simulink model "InvPend"  (Simulink 7.6)
settings: Solver=ode4  StartTime=0.0  StopTime=20  FixedStep=0.01  RelTol=1e-3
values from neighbouring files (symbols this model uses):
  c = 6/(7*l + (b^2)/l)    (= 1.71389396709)    [MasterP_4DInvPendData_BEST.m]    (also in MasterP_4DInvPendData_MAIN.m)
  g = 9.81    [MasterP_4DInvPendData_BEST.m]    (also in MasterP_4DInvPendData_MAIN.m)
  kP = 1    [MasterP_4DInvPendData_BEST.m]    (also in MasterP_4DInvPendData_MAIN.m)
  T1 = 0.0395    [MasterP_4DInvPendData_BEST.m]    (also in MasterP_4DInvPendData_MAIN.m)
undefined symbols (not defined in the file or in its folder): SU
settings Model: Creator=Mohsen  LastModifiedBy=Mohsen

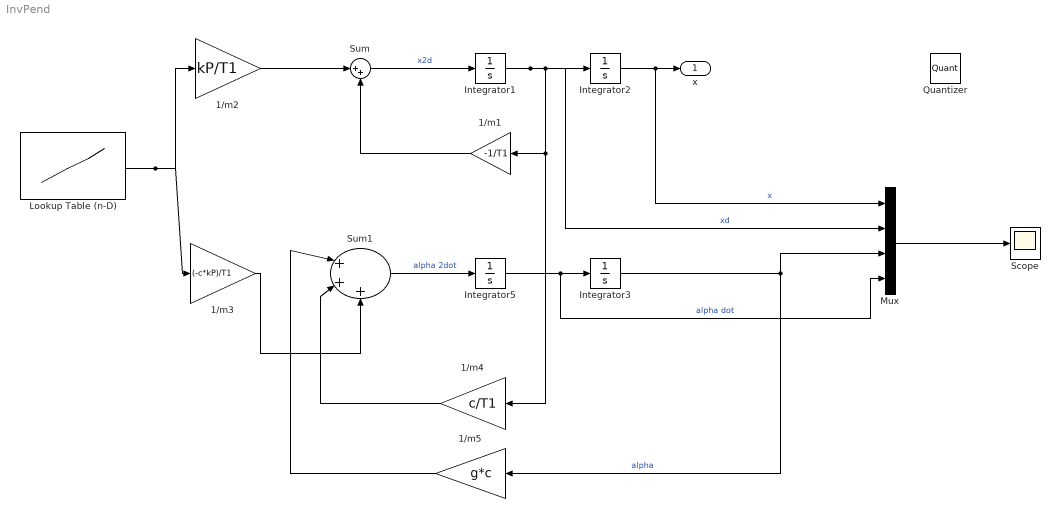
== system InvPend ==
  1/m1 : Gain  Gain=-1/T1
  1/m2 : Gain  Gain=kP/T1
  1/m3 : Gain  Gain=(-c*kP)/T1
  1/m4 : Gain  Gain=c/T1
  1/m5 : Gain  Gain=g*c
  Integrator1 : Integrator  InitialCondition=1
  Integrator2 : Integrator  InitialCondition=0.02
  Integrator3 : Integrator  InitialCondition=10
  Integrator5 : Integrator  InitialCondition=10
  Lookup Table (n-D) : Lookup_n-D  NumberOfTableDimensions=4  BreakpointsForDimension1=[-4:1:4]  BreakpointsForDimension2=[-4:1:4]  BreakpointsForDimension3=[(-pi):(pi/4):(pi)]  BreakpointsForDimension4=[(-2*pi):(pi/2):(2*pi)]  Table=SU  RndMeth=Zero  InputSameDT=on
  Mux : Mux
  Quantizer : Quantizer  QuantizationInterval=1
  Scope : Scope
      settings: TimeRange=20  YMin=-20  YMax=10  SaveName=states  DataFormat=Array
  Sum : Sum  Inputs=|++
  Sum1 : Sum  Inputs=|+++
  x : Outport
  wires:
  Mux/1 -> Scope/1
  Integrator1/1 -> Integrator2/1, 1/m1/1, 1/m4/1, Mux/2  "xd"
  Integrator2/1 -> x/1, Mux/1  "x"
  1/m1/1 -> Sum/2
  Sum/1 -> Integrator1/1  "x2d"
  1/m2/1 -> Sum/1
  Integrator3/1 -> 1/m5/1, Mux/3  "alpha"
  Sum1/1 -> Integrator5/1  "alpha 2dot"
  1/m3/1 -> Sum1/3
  Lookup Table (n-D)/1 -> 1/m2/1, 1/m3/1
  1/m4/1 -> Sum1/2
  1/m5/1 -> Sum1/1
  Integrator5/1 -> Integrator3/1, Mux/4  "alpha dot"
